simulink subsystem "Inner_loop"  (R2024a)
settings: Solver=VariableStepAuto  StartTime=0.0  StopTime=10.0  RelTol=1e-3
undefined symbols (not defined in the file): DiscIntNeverNeededParam
libraries: simulink x2
settings Model: Creator=gurt1  LastModifiedBy=gurt1
settings RTWCC: GPUComputeCapability=3.5

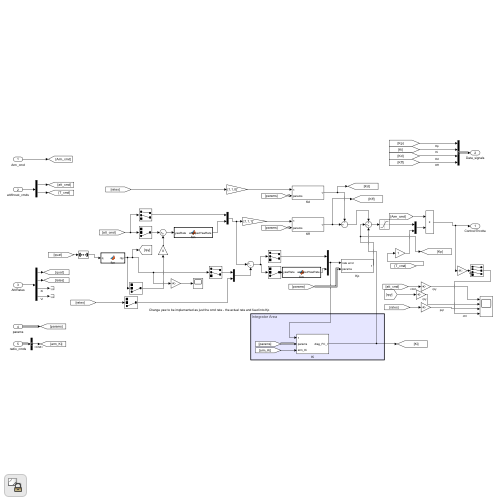
[thumbnail: Simulink's stored preview of the top-level diagram]
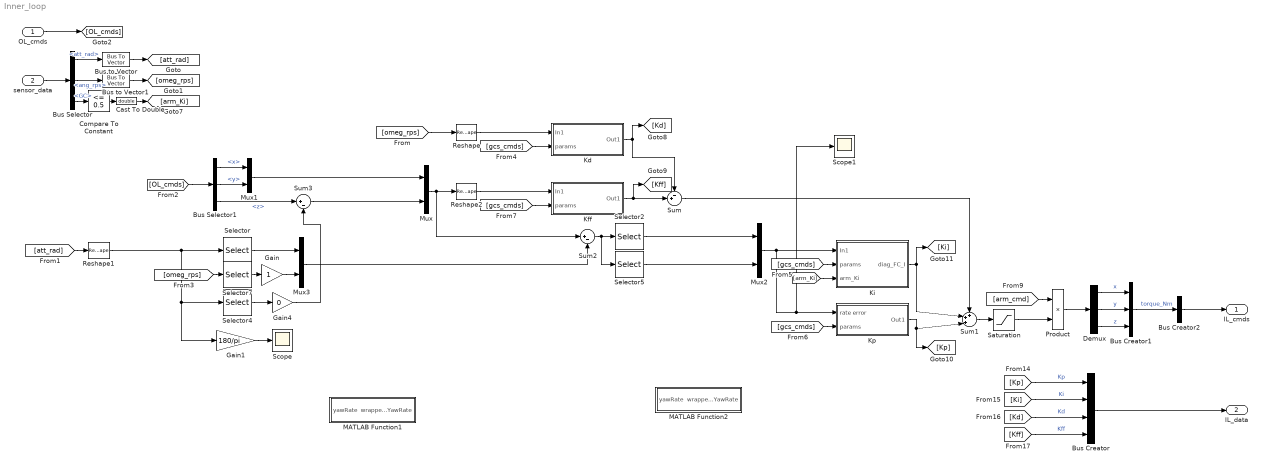
== system Inner_loop ==
  OL_cmds : Inport
  sensor_data : Inport  Port=2
  Bus Creator : BusCreator  Inputs=4
  Bus Creator1 : BusCreator  Inputs=3
  Bus Creator2 : BusCreator  Inputs=1
  Bus Selector : BusSelector  OutputSignals=att_rad,ang_rps,flags.GC
  Bus Selector1 : BusSelector  OutputSignals=att_rad.x,att_rad.y,ang_rps.z
  Bus to Vector : BusToVector
  Bus to Vector1 : BusToVector
  Cast To Double : DataTypeConversion  OutDataTypeStr=double  SaturateOnIntegerOverflow=off  RndMeth=Floor
  Compare To Constant : simulink/Logic and Bit Operations/Compare To Constant  relop=<=  const=0.5  OutDataTypeStr=boolean
  Demux : Demux  Outputs=3
  Gain : Gain
  Gain1 : Gain  Gain=180/pi
  Gain4 : Gain  Gain=0
  Kd : Subsystem
  Kff : Subsystem
  Ki : Subsystem
  Kp : Subsystem
  MATLAB Function1 : MATLAB Function  TreatAsAtomicUnit=on
  MATLAB Function2 : MATLAB Function  TreatAsAtomicUnit=on
  Mux{,1..3} (4 alike) : Mux  Inputs=2
  Product : Product
  Reshape : Reshape
  Reshape1 : Reshape
  Reshape2 : Reshape
  Saturation : Saturate  UpperLimit=2*pi  LowerLimit=-2*pi
  Scope : Scope
  Scope1 : Scope
  Selector : Selector  InputPortWidth=3  IndexOptions=Index vector (dialog)  Indices=[1 2]  OutputSizes=1
  Selector2 : Selector  InputPortWidth=3  IndexOptions=Index vector (dialog)  Indices=[1,2]  OutputSizes=1
  Selector4 : Selector  InputPortWidth=3  IndexOptions=Index vector (dialog)  Indices=[3]  OutputSizes=1
  Selector5 : Selector  InputPortWidth=3  IndexOptions=Index vector (dialog)  Indices=[3]  OutputSizes=1
  Selector7 : Selector  InputPortWidth=3  IndexOptions=Index vector (dialog)  Indices=[3]  OutputSizes=1
  Sum : Sum  Inputs=-+|
  Sum1 : Sum  Inputs=+++|
  Sum2 : Sum  Inputs=|+-
  Sum3 : Sum  Inputs=|+-
  IL_cmds : Outport
  IL_data : Outport  Port=2
  wires:
  [gcs_cmds] -> Ki/2(params)
  [att_rad] -> Reshape1/1
  [arm_Ki] -> Ki/3(arm_Ki)
  Ki/1(diag_FC_I) -> Sum1/2, [Ki]
  [Kp] -> Bus Creator/1  "Kp"
  Gain4/1 -> Sum3/2
  [Ki] -> Bus Creator/2  "Ki"
  Mux/1 -> Sum2/1, Reshape2/1
  [Kd] -> Bus Creator/3  "Kd"
  Sum2/1 -> Selector2/1, Selector5/1
  [Kff] -> Bus Creator/4  "Kff"
  Selector4/1 -> Gain4/1
  OL_cmds/1 -> [OL_cmds]
  Bus Selector/1 -> Bus to Vector/1  "<att_rad>"
  Bus Selector/2 -> Bus to Vector1/1  "<ang_rps>"
  Bus Creator/1 -> IL_data/1
  [omeg_rps] -> Selector7/1
  Reshape1/1 -> Selector/1, Selector4/1, Gain1/1
  Mux3/1 -> Sum2/2
  Selector/1 -> Mux3/1
  Kp/1(Out1) -> [Kp], Sum1/3
  Mux2/1 -> Scope1/1, Kp/1(rate error), Ki/1(In1)
  Gain1/1 -> Scope/1
  Mux1/1 -> Mux/1
  [gcs_cmds] -> Kp/2(params)
  Sum3/1 -> Mux/2
  [omeg_rps] -> Reshape/1
  Reshape/1 -> Kd/1(In1)
  [gcs_cmds] -> Kd/2(params)
  Reshape2/1 -> Kff/1(In1)
  Selector2/1 -> Mux2/1
  [gcs_cmds] -> Kff/2(params)
  Kd/1(Out1) -> Sum/1, [Kd]
  Kff/1(Out1) -> [Kff], Sum/2
  Sum/1 -> Sum1/1
  [arm_cmd] -> Product/1
  Selector5/1 -> Mux2/2
  Sum1/1 -> Saturation/1
  Saturation/1 -> Product/2
  sensor_data/1 -> Bus Selector/1
  Bus to Vector/1 -> [att_rad]
  Bus to Vector1/1 -> [omeg_rps]
  Bus Selector/3 -> Compare To Constant/1  "<GC>"
  Compare To Constant/1 -> Cast To Double/1
  Cast To Double/1 -> [arm_Ki]
  [OL_cmds] -> Bus Selector1/1
  Bus Selector1/1 -> Mux1/1  "<x>"
  Bus Selector1/2 -> Mux1/2  "<y>"
  Bus Selector1/3 -> Sum3/1  "<z>"
  Product/1 -> Demux/1
  Demux/1 -> Bus Creator1/1  "x"
  Demux/2 -> Bus Creator1/2  "y"
  Demux/3 -> Bus Creator1/3  "z"
  Bus Creator1/1 -> Bus Creator2/1  "torque_Nm"
  Bus Creator2/1 -> IL_cmds/1
  Selector7/1 -> Gain/1
  Gain/1 -> Mux3/2

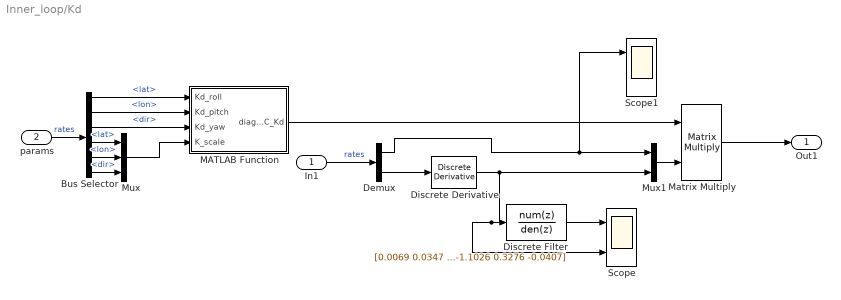
== system Inner_loop/Kd ==
  In1 : Inport
  params : Inport  Port=2
  Bus Selector : BusSelector  OutputSignals=IL.kd.lat,IL.kd.lon,IL.kd.dir,IL.scale.lat,IL.scale.lon,IL.scale.dir
  Demux : Demux  Outputs=[2 1]
  Discrete Derivative : simulink/Discrete/Discrete Derivative  gainval=1.0  ICPrevScaledInput=0.0  OutMin=[]  OutMax=[]  OutDataType=fixdt(1, 16)  OutScaling=2^-10  DoSatur=off
  Discrete Filter : DiscreteFilter  Numerator=[0.0069 0.0347 0.0693 0.0693 0.0347 0.0069]  Denominator=[1 -1.9759 2.0135 -1.1026 0.3276 -0.0407]
  MATLAB Function : MATLAB Function  TreatAsAtomicUnit=on
  Matrix Multiply : Product  Multiplication=Matrix(*)
  Mux : Mux  Inputs=3
  Mux1 : Mux  Inputs=2
  Scope : Scope  NumInputPorts=2
  Scope1 : Scope  NumInputPorts=2
  Out1 : Outport
  wires:
  Demux/1 -> Mux1/1, Scope1/1
  Discrete Filter/1 -> Scope/1
  Discrete Derivative/1 -> Discrete Filter/1, Scope/2, Mux1/2
  Demux/2 -> Discrete Derivative/1
  Mux1/1 -> Matrix Multiply/2
  In1/1 -> Demux/1  "rates"
  Mux/1 -> MATLAB Function/4(K_scale)
  Bus Selector/6 -> Mux/3  "<dir>"
  Bus Selector/5 -> Mux/2  "<lon>"
  Bus Selector/4 -> Mux/1  "<lat>"
  MATLAB Function/1(diag_FC_Kd) -> Matrix Multiply/1
  Bus Selector/3 -> MATLAB Function/3(Kd_yaw)  "<dir>"
  Bus Selector/1 -> MATLAB Function/1(Kd_roll)  "<lat>"
  Bus Selector/2 -> MATLAB Function/2(Kd_pitch)  "<lon>"
  params/1 -> Bus Selector/1  "rates"
  Matrix Multiply/1 -> Out1/1

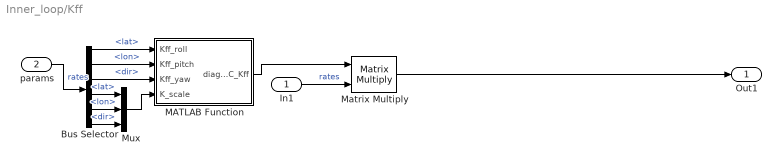
== system Inner_loop/Kff ==
  In1 : Inport
  params : Inport  Port=2
  Bus Selector : BusSelector  OutputSignals=IL.kff.lat,IL.kff.lon,IL.kff.dir,IL.scale.lat,IL.scale.lon,IL.scale.dir
  MATLAB Function : MATLAB Function  TreatAsAtomicUnit=on
  Matrix Multiply : Product  Multiplication=Matrix(*)
  Mux : Mux  Inputs=3
  Out1 : Outport
  wires:
  Mux/1 -> MATLAB Function/4(K_scale)
  Bus Selector/6 -> Mux/3  "<dir>"
  Bus Selector/5 -> Mux/2  "<lon>"
  Bus Selector/4 -> Mux/1  "<lat>"
  MATLAB Function/1(diag_FC_Kff) -> Matrix Multiply/1
  Bus Selector/3 -> MATLAB Function/3(Kff_yaw)  "<dir>"
  params/1 -> Bus Selector/1  "rates"
  Bus Selector/2 -> MATLAB Function/2(Kff_pitch)  "<lon>"
  Bus Selector/1 -> MATLAB Function/1(Kff_roll)  "<lat>"
  In1/1 -> Matrix Multiply/2  "rates"
  Matrix Multiply/1 -> Out1/1

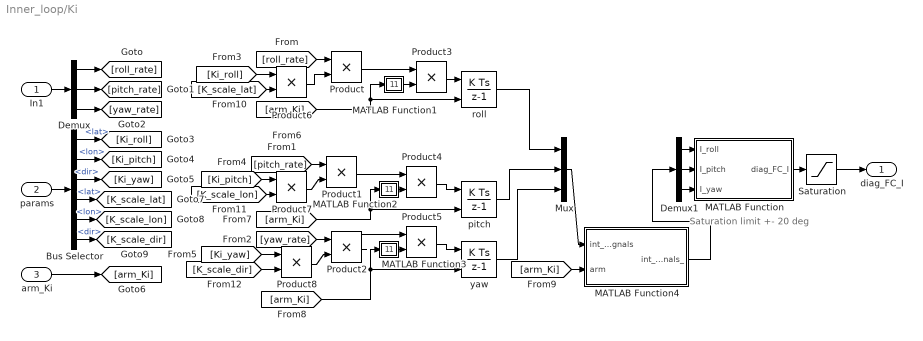
== system Inner_loop/Ki ==
  note: Saturation limit +- 20 deg
  In1 : Inport
  params : Inport  Port=2
  arm_Ki : Inport  Port=3
  Bus Selector : BusSelector  OutputSignals=IL.ki.lat,IL.ki.lon,IL.ki.dir,IL.scale.lat,IL.scale.lon,IL.scale.dir
  Demux : Demux  Outputs=3
  Demux1 : Demux  Outputs=3
  MATLAB Function : MATLAB Function  TreatAsAtomicUnit=on
  MATLAB Function1 : MATLAB Function  TreatAsAtomicUnit=on
  MATLAB Function2 : MATLAB Function  TreatAsAtomicUnit=on
  MATLAB Function3 : MATLAB Function  TreatAsAtomicUnit=on
  MATLAB Function4 : MATLAB Function  TreatAsAtomicUnit=on
  Mux : Mux  Inputs=3
  Product{,1..8} (9 alike) : Product
  Saturation : Saturate  UpperLimit=20*(pi/180)  LowerLimit=-20*(pi/180)
  pitch : DiscreteIntegrator  ExternalReset=either  SampleTime=-1  ICPrevOutput=DiscIntNeverNeededParam  ICPrevScaledInput=DiscIntNeverNeededParam
  roll : DiscreteIntegrator  ExternalReset=either  SampleTime=-1  ICPrevOutput=DiscIntNeverNeededParam  ICPrevScaledInput=DiscIntNeverNeededParam
  yaw : DiscreteIntegrator  ExternalReset=either  SampleTime=-1  ICPrevOutput=DiscIntNeverNeededParam  ICPrevScaledInput=DiscIntNeverNeededParam
  diag_FC_I : Outport
  wires:
  Product8/1 -> Product2/2
  [K_scale_dir] -> Product8/2
  [Ki_yaw] -> Product8/1
  Product7/1 -> Product1/2
  [K_scale_lon] -> Product7/2
  [Ki_pitch] -> Product7/1
  Product6/1 -> Product/2
  [K_scale_lat] -> Product6/2
  Bus Selector/6 -> [K_scale_dir]  "<dir>"
  Bus Selector/5 -> [K_scale_lon]  "<lon>"
  Bus Selector/4 -> [K_scale_lat]  "<lat>"
  [Ki_roll] -> Product6/1
  [arm_Ki] -> MATLAB Function4/2(arm)
  MATLAB Function4/1(int_signals_) -> Demux1/1
  Demux1/3 -> MATLAB Function/3(I_yaw)
  Demux1/2 -> MATLAB Function/2(I_pitch)
  Demux1/1 -> MATLAB Function/1(I_roll)
  Mux/1 -> MATLAB Function4/1(int_signals)
  Saturation/1 -> diag_FC_I/1
  MATLAB Function3/1(arm_val) -> Product5/2
  MATLAB Function2/1(arm_val) -> Product4/2
  Product/1 -> Product3/1
  MATLAB Function1/1(arm_val) -> Product3/2
  Product5/1 -> yaw/1
  [arm_Ki] -> yaw/2, MATLAB Function3/1(arm)
  Product2/1 -> Product5/1
  Product4/1 -> pitch/1
  Product1/1 -> Product4/1
  Product3/1 -> roll/1
  MATLAB Function/1(diag_FC_I) -> Saturation/1
  yaw/1 -> Mux/3
  pitch/1 -> Mux/2
  roll/1 -> Mux/1
  [arm_Ki] -> MATLAB Function2/1(arm), pitch/2
  [arm_Ki] -> roll/2, MATLAB Function1/1(arm)
  arm_Ki/1 -> [arm_Ki]
  Bus Selector/3 -> [Ki_yaw]  "<dir>"
  Bus Selector/2 -> [Ki_pitch]  "<lon>"
  Bus Selector/1 -> [Ki_roll]  "<lat>"
  [yaw_rate] -> Product2/1
  [pitch_rate] -> Product1/1
  [roll_rate] -> Product/1
  Demux/3 -> [yaw_rate]
  Demux/2 -> [pitch_rate]
  Demux/1 -> [roll_rate]
  In1/1 -> Demux/1
  params/1 -> Bus Selector/1

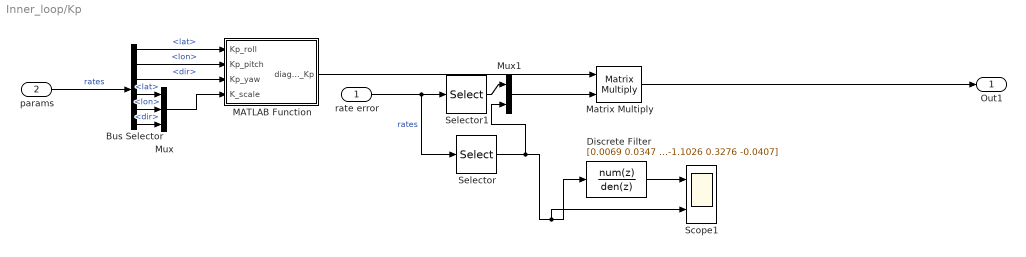
== system Inner_loop/Kp ==
  rate error : Inport
  params : Inport  Port=2
  Bus Selector : BusSelector  OutputSignals=IL.kp.lat,IL.kp.lon,IL.kp.dir,IL.scale.lat,IL.scale.lon,IL.scale.dir
  Discrete Filter : DiscreteFilter  Numerator=[0.0069 0.0347 0.0693 0.0693 0.0347 0.0069]  Denominator=[1 -1.9759 2.0135 -1.1026 0.3276 -0.0407]
  MATLAB Function : MATLAB Function  TreatAsAtomicUnit=on
  Matrix Multiply : Product  Multiplication=Matrix(*)
  Mux : Mux  Inputs=3
  Mux1 : Mux  Inputs=[2 1]
  Scope1 : Scope  NumInputPorts=2
  Selector : Selector  InputPortWidth=3  IndexOptions=Index vector (dialog)  Indices=[3]  OutputSizes=1
  Selector1 : Selector  InputPortWidth=3  IndexOptions=Index vector (dialog)  Indices=[1 2]  OutputSizes=1
  Out1 : Outport
  wires:
  Selector1/1 -> Mux1/1
  Mux1/1 -> Matrix Multiply/2
  Discrete Filter/1 -> Scope1/1
  Selector/1 -> Scope1/2, Discrete Filter/1, Mux1/2
  rate error/1 -> Selector/1, Selector1/1  "rates"
  Mux/1 -> MATLAB Function/4(K_scale)
  Bus Selector/6 -> Mux/3  "<dir>"
  Bus Selector/5 -> Mux/2  "<lon>"
  Bus Selector/4 -> Mux/1  "<lat>"
  params/1 -> Bus Selector/1  "rates"
  Bus Selector/2 -> MATLAB Function/2(Kp_pitch)  "<lon>"
  Bus Selector/1 -> MATLAB Function/1(Kp_roll)  "<lat>"
  Bus Selector/3 -> MATLAB Function/3(Kp_yaw)  "<dir>"
  MATLAB Function/1(diag_FC_Kp) -> Matrix Multiply/1
  Matrix Multiply/1 -> Out1/1

== matlab function Inner_loop/Kd/MATLAB Function ==
  data: Kd_roll input; diag_FC_Kd output; Kd_pitch input; Kd_yaw input; K_scale input
function diag_FC_Kd = fcn(Kd_roll, Kd_pitch, Kd_yaw, K_scale)

diag_FC_Kd = [Kd_roll 0 0; 0 Kd_pitch 0; 0 0 Kd_yaw];

diag_K_scale = [K_scale(1) 0 0; 0 K_scale(2) 0; 0 0 K_scale(3)];

diag_FC_Kd = diag_FC_Kd.*diag_K_scale;

== matlab function Inner_loop/Kff/MATLAB Function ==
  data: Kff_roll input; diag_FC_Kff output; Kff_pitch input; Kff_yaw input; K_scale input
function diag_FC_Kff = fcn(Kff_roll, Kff_pitch, Kff_yaw, K_scale)

diag_FC_Kff = [Kff_roll 0 0; 0 Kff_pitch 0; 0 0 Kff_yaw];

diag_K_scale = [K_scale(1) 0 0; 0 K_scale(2) 0; 0 0 K_scale(3)];

diag_FC_Kff = diag_FC_Kff.*diag_K_scale;

== matlab function Inner_loop/Ki/MATLAB Function ==
  data: I_roll input; diag_FC_I output; I_pitch input; I_yaw input
function diag_FC_I = fcn(I_roll, I_pitch, I_yaw)

diag_FC_I = [I_roll; I_pitch; I_yaw];

== matlab function Inner_loop/Ki/MATLAB Function1 ==
  data: arm input; arm_val output
function arm_val = fcn(arm)

if arm == 1
    arm_val = 1;
elseif arm == 2
    arm_val = 0;
else
    arm_val = 1;
end

== matlab function Inner_loop/Ki/MATLAB Function2 ==
  data: arm input; arm_val output
function arm_val = fcn(arm)

if arm == 1
    arm_val = 1;
elseif arm == 2
    arm_val = 0;
else
    arm_val = 1;
end

== matlab function Inner_loop/Ki/MATLAB Function3 ==
  data: arm input; arm_val output
function arm_val = fcn(arm)

if arm == 1
    arm_val = 1;
elseif arm == 2
    arm_val = 0;
else
    arm_val = 1;
end

== matlab function Inner_loop/Kp/MATLAB Function ==
  data: Kp_roll input; diag_FC_Kp output; Kp_pitch input; Kp_yaw input; K_scale input
function diag_FC_Kp = fcn(Kp_roll, Kp_pitch, Kp_yaw, K_scale)

diag_FC_Kp = [Kp_roll 0 0; 0 Kp_pitch 0; 0 0 Kp_yaw];

diag_K_scale = [K_scale(1) 0 0; 0 K_scale(2) 0; 0 0 K_scale(3)];

diag_FC_Kp = diag_FC_Kp.*diag_K_scale;

== matlab function Inner_loop/MATLAB Function1 ==
  data: yawRate input; wrappedYawRate output
function wrappedYawRate = fcn(yawRate)
    % Define the bounds for wrapping
    lowerBound = -2*pi;
    upperBound = 2*pi;
    
    % Wrap the yaw rate using modulo
    wrappedYawRate = mod(yawRate - lowerBound, upperBound - lowerBound) + lowerBound;
    
    % Ensure the result is wrapped
    if wrappedYawRate > upperBound
        wrappedYawRate = wrappedYawRate - 2*pi;
    elseif wrappedYawRate < lowerBound
        wrappedYawRate = wrappedYawRate + 2*pi;
    end
end

== matlab function Inner_loop/MATLAB Function2 ==
  data: yawRate input; wrappedYawRate output
function wrappedYawRate = fcn(yawRate)
    % Define the bounds for wrapping
    lowerBound = -2*pi;
    upperBound = 2*pi;
    
    % Wrap the yaw rate using modulo
    wrappedYawRate = mod(yawRate - lowerBound, upperBound - lowerBound) + lowerBound;
    
    % Ensure the result is wrapped
    if wrappedYawRate > upperBound
        wrappedYawRate = wrappedYawRate - 2*pi;
    elseif wrappedYawRate < lowerBound
        wrappedYawRate = wrappedYawRate + 2*pi;
    end
end

== matlab function Inner_loop/Ki/MATLAB Function4 ==
  data: int_signals input; int_signals_ output; arm input
function int_signals_ = integrator_catch(int_signals,arm)


if arm == 2
    int_signals_ = int_signals*0;
else
    int_signals_ = int_signals;
end
